simulink library "mlp_mid_level_processor_lib"  (R2015b)
settings: Solver=ode45  StartTime=0.0  StopTime=10.0  RelTol=1e-3
undefined symbols (not defined in the file or in its folder): cmc_mode_cmd, cmc_state_cmd_a, cmc_state_cmd_b, localization_mode_cmd, speed_gain_cmd
libraries: cmc_command_and_mode_control x1, cvs_computer_vision_system_lib x1
settings Model: Creator=rhnakamu  LastModifiedBy=jfusco1
settings DataIOCC: SaveFormat=Array
settings HardwareCC: ProdBitPerPointer=32  ProdLargestAtomicFloat=None  ProdIntDivRoundTo=Undefined  ProdEndianess=Unspecified  ProdWordSize=32  ProdHWDeviceType=32-bit Generic
settings GRTTargetCC: GeneratePreprocessorConditionals=Disable all
settings ConfigComp: CovModelRefEnable=Off

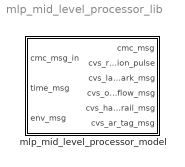
== system mlp_mid_level_processor_lib ==
  mlp_mid_level_processor_model : Subsystem

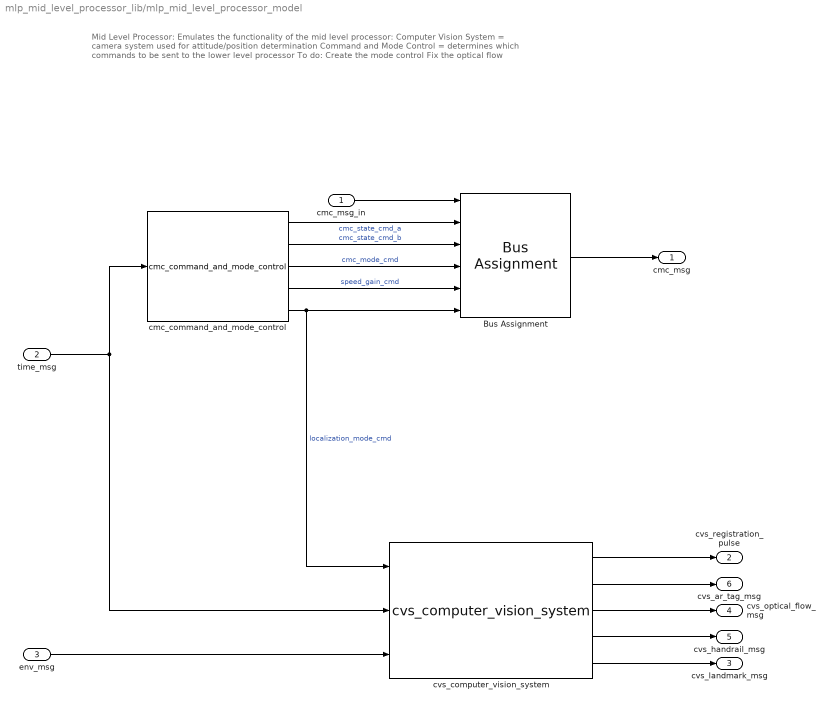
== system mlp_mid_level_processor_lib/mlp_mid_level_processor_model ==
  note: Mid Level Processor:
      | Emulates the functionality of the mid level processor:
      | Computer Vision System = camera system used for attitude/position determination
      | Command and Mode Control = determines which commands to be sent to the lower level processor
      |
      | To do:
      | Create the mode control
      | Fix the optical flow
  cmc_msg_in : Inport  OutDataTypeStr=Bus: cmc_msg
  time_msg : Inport  Port=2
  env_msg : Inport  Port=3  OutDataTypeStr=Bus: env_msg
  Bus Assignment : BusAssignment  AssignedSignals=cmc_state_cmd_a,cmc_state_cmd_b,cmc_mode_cmd,speed_gain_cmd,localization_mode_cmd
  cmc_command_and_mode_control : cmc_command_and_mode_control/cmc_command_and_mode_control
  cvs_computer_vision_system : cvs_computer_vision_system_lib/cvs_computer_vision_system
  cmc_msg : Outport  OutDataTypeStr=Bus: cmc_msg
  cvs_registration_pulse : Outport  Port=2
  cvs_landmark_msg : Outport  Port=3
  cvs_optical_flow_msg : Outport  Port=4
  cvs_handrail_msg : Outport  Port=5
  cvs_ar_tag_msg : Outport  Port=6
  wires:
  cvs_computer_vision_system/4 -> cvs_handrail_msg/1
  cvs_computer_vision_system/1 -> cvs_registration_pulse/1
  env_msg/1 -> cvs_computer_vision_system/3
  cmc_command_and_mode_control/1 -> Bus Assignment/2  "cmc_state_cmd_a"
  cmc_command_and_mode_control/3 -> Bus Assignment/4  "cmc_mode_cmd"
  cmc_command_and_mode_control/2 -> Bus Assignment/3  "cmc_state_cmd_b"
  cvs_computer_vision_system/3 -> cvs_optical_flow_msg/1
  time_msg/1 -> cmc_command_and_mode_control/1, cvs_computer_vision_system/2
  cmc_command_and_mode_control/5 -> cvs_computer_vision_system/1, Bus Assignment/6  "localization_mode_cmd"
  cmc_command_and_mode_control/4 -> Bus Assignment/5  "speed_gain_cmd"
  cvs_computer_vision_system/5 -> cvs_landmark_msg/1
  cvs_computer_vision_system/2 -> cvs_ar_tag_msg/1
  cmc_msg_in/1 -> Bus Assignment/1
  Bus Assignment/1 -> cmc_msg/1
